simulink model "EngineCtrl_V1_1"  (R2018a)
settings: Solver=VariableStepAuto  StartTime=0.0  StopTime=10.0  FixedStep=sampletime  RelTol=1e-3  EnableMultiTasking=on
PreLoadFcn:
  | EngineCtrl_V1_BusInfo
libraries: simulink x2, simulink_extras x1
settings Model: Creator=IAEC nishito  LastModifiedBy=E00026
settings DataIOCC: LimitDataPoints=on  SaveFormat=Array  SignalLoggingSaveFormat=ModelDataLogs  SaveOutput=off  SaveTime=off
settings OptimizationCC: DefaultParameterBehavior=Inlined  ExpressionDepthLimit=2147483647  LifeSpan=inf
settings DebuggingCC: SolverPrmCheckMsg=warning  FcnCallInpInsideContextMsg=warning  StateNameClashWarn=warning  SFUnexpectedBacktrackingDiag=warning  SFNoUnconditionalDefaultTransitionDiag=warning  SFExecutionAtInitializationDiag=none
settings HardwareCC: ProdBitPerPointer=32  ProdBitPerSizeT=32  ProdBitPerPtrDiffT=32  ProdLargestAtomicFloat=None  ProdIntDivRoundTo=Undefined  ProdEndianess=Unspecified  ProdWordSize=32  ProdHWDeviceType=32-bit Generic
settings ModelReferenceCC: UpdateModelReferenceTargets=IfOutOfDate  PropagateSignalLabelsOutOfModel=off
settings CodeAppCC: StateflowObjectComments=on
settings GRTTargetCC: TargetLangStandard=C89/C90 (ANSI)  GeneratePreprocessorConditionals=Disable all  CombineOutputUpdateFcns=off  GRTInterface=on
settings ConfigComp: CovMetricSettings=dw  CovHtmlReporting=on  CovSaveCumulativeToWorkspaceVar=on  CovSaveSingleToWorkspaceVar=on  CovExternalEMLEnable=off

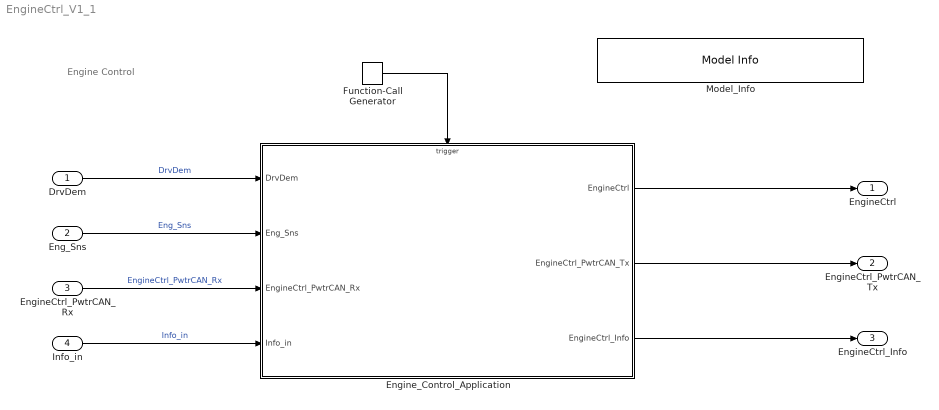
== system EngineCtrl_V1_1 ==
  note: Engine Control
  DrvDem : Inport  OutDataTypeStr=Bus: Driver_demand_Bus
      settings: AttributesFormatString=%<OutDataTypeStr>
  Eng_Sns : Inport  Port=2  OutDataTypeStr=Bus: Engine_sensor_Bus
      settings: AttributesFormatString=%<OutDataTypeStr>
  EngineCtrl_PwtrCAN_Rx : Inport  Port=3  OutDataTypeStr=Bus: EngineCtrl_PwtrCAN_Rx_Bus
      settings: AttributesFormatString=<%<OutDataTypeStr>>
  Info_in : Inport  Port=4  OutDataTypeStr=Bus: EngineCtrl_Info_in_Bus
      settings: AttributesFormatString=%<OutDataTypeStr>
  Engine_Control_Application : Subsystem
  Function-Call Generator : simulink/Ports & Subsystems/Function-Call Generator  sample_time=0.01  numberOfIterations=1
      settings: AttributesFormatString=<sample_time=%<sample_time>>
  Model_Info : simulink/Model-Wide Utilities/Model Info  Frame=on  DisplayStringWithTags=|  HorizontalTextAlignment=Left  LeftAlignmentValue=0.02
      | Version  %<ModelVersion>
      | LastModifided by %<LastModifiedBy>  Date %<LastModificationDate>
      | Description  %<Description>
  EngineCtrl : Outport  OutDataTypeStr=Bus: EngineCtrl_Bus
      settings: AttributesFormatString=<%<OutDataTypeStr>>
  EngineCtrl_PwtrCAN_Tx : Outport  Port=2  OutDataTypeStr=Bus: EngineCtrl_PwtrCAN_Tx_Bus
      settings: AttributesFormatString=<%<OutDataTypeStr>>
  EngineCtrl_Info : Outport  Port=3  OutDataTypeStr=Bus: EngineCtrl_Info_Bus
      settings: AttributesFormatString=<%<OutDataTypeStr>>
  wires:
  EngineCtrl_PwtrCAN_Rx/1 -> Engine_Control_Application/3(EngineCtrl_PwtrCAN_Rx)  "EngineCtrl_PwtrCAN_Rx"
  DrvDem/1 -> Engine_Control_Application/1(DrvDem)  "DrvDem"
  Eng_Sns/1 -> Engine_Control_Application/2(Eng_Sns)  "Eng_Sns"
  Function-Call Generator/1 -> Engine_Control_Application/Trigger
  Engine_Control_Application/2(EngineCtrl_PwtrCAN_Tx) -> EngineCtrl_PwtrCAN_Tx/1
  Engine_Control_Application/1(EngineCtrl) -> EngineCtrl/1
  Engine_Control_Application/3(EngineCtrl_Info) -> EngineCtrl_Info/1
  Info_in/1 -> Engine_Control_Application/4(Info_in)  "Info_in"

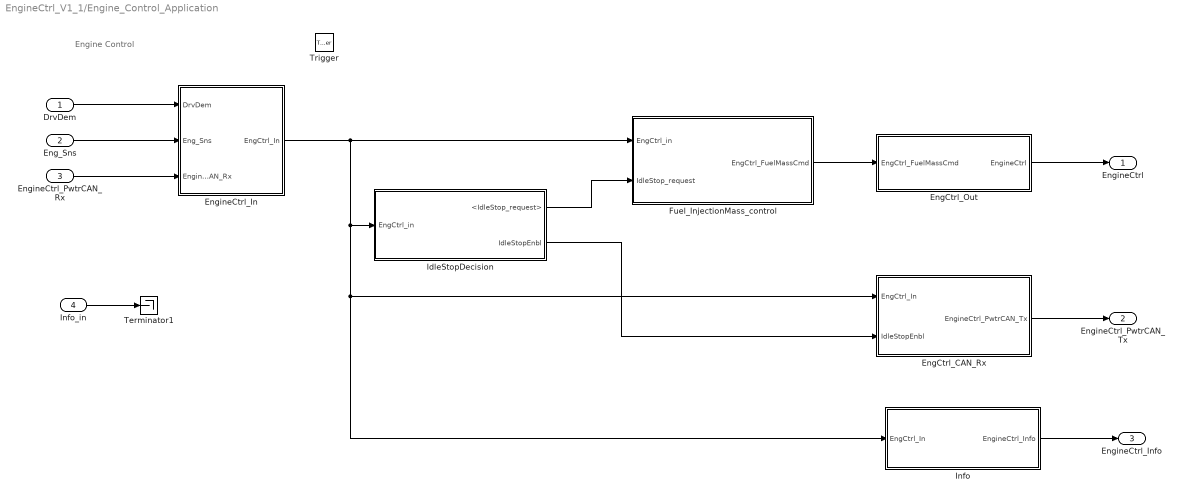
== system EngineCtrl_V1_1/Engine_Control_Application ==
  note: Engine Control
  DrvDem : Inport
  Eng_Sns : Inport  Port=2
  EngineCtrl_PwtrCAN_Rx : Inport  Port=3
  Info_in : Inport  Port=4
  Trigger : TriggerPort  TriggerType=function-call  VariantControl=Variant  PortDimensions=1
  EngCtrl_CAN_Rx : Subsystem
  EngCtrl_Out : Subsystem
  EngineCtrl_In : Subsystem
  Fuel_InjectionMass_control : Subsystem
  IdleStopDecision : Subsystem
  Info : Subsystem
  Terminator1 : Terminator
  EngineCtrl : Outport
  EngineCtrl_PwtrCAN_Tx : Outport  Port=2
  EngineCtrl_Info : Outport  Port=3
  wires:
  DrvDem/1 -> EngineCtrl_In/1(DrvDem)
  Info_in/1 -> Terminator1/1
  EngCtrl_CAN_Rx/1(EngineCtrl_PwtrCAN_Tx) -> EngineCtrl_PwtrCAN_Tx/1
  IdleStopDecision/2(IdleStopEnbl) -> EngCtrl_CAN_Rx/2(IdleStopEnbl)
  Eng_Sns/1 -> EngineCtrl_In/2(Eng_Sns)
  EngineCtrl_PwtrCAN_Rx/1 -> EngineCtrl_In/3(EngineCtrl_PwtrCAN_Rx)
  EngineCtrl_In/1(EngCtrl_In) -> Info/1(EngCtrl_In), EngCtrl_CAN_Rx/1(EngCtrl_In), IdleStopDecision/1(EngCtrl_in), Fuel_InjectionMass_control/1(EngCtrl_in)
  Info/1(EngineCtrl_Info) -> EngineCtrl_Info/1
  Fuel_InjectionMass_control/1(EngCtrl_FuelMassCmd) -> EngCtrl_Out/1(EngCtrl_FuelMassCmd)
  EngCtrl_Out/1(EngineCtrl) -> EngineCtrl/1
  IdleStopDecision/1(<IdleStop_request>) -> Fuel_InjectionMass_control/2(IdleStop_request)

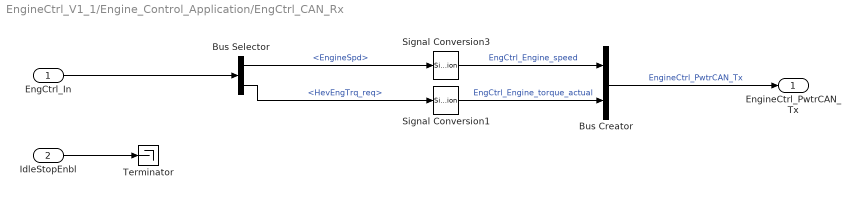
== system EngineCtrl_V1_1/Engine_Control_Application/EngCtrl_CAN_Rx ==
  EngCtrl_In : Inport
  IdleStopEnbl : Inport  Port=2
  Bus Creator : BusCreator  Inputs=2  OutDataTypeStr=Bus: EngineCtrl_PwtrCAN_Tx_Bus
      settings: AttributesFormatString=%<OutDataTypeStr>
  Bus Selector : BusSelector  OutputSignals=EngineSpd,HevEngTrq_req
  Signal Conversion1 : SignalConversion  OverrideOpt=off
  Signal Conversion3 : SignalConversion  OverrideOpt=off
  Terminator : Terminator
  EngineCtrl_PwtrCAN_Tx : Outport
  wires:
  Bus Creator/1 -> EngineCtrl_PwtrCAN_Tx/1  "EngineCtrl_PwtrCAN_Tx"
  Signal Conversion3/1 -> Bus Creator/1  "EngCtrl_Engine_speed"
  Signal Conversion1/1 -> Bus Creator/2  "EngCtrl_Engine_torque_actual"
  EngCtrl_In/1 -> Bus Selector/1
  Bus Selector/1 -> Signal Conversion3/1  "<EngineSpd>"
  Bus Selector/2 -> Signal Conversion1/1  "<HevEngTrq_req>"
  IdleStopEnbl/1 -> Terminator/1

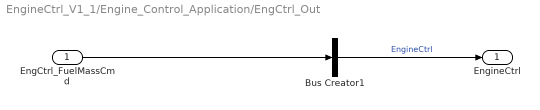
== system EngineCtrl_V1_1/Engine_Control_Application/EngCtrl_Out ==
  EngCtrl_FuelMassCmd : Inport
  Bus Creator1 : BusCreator  Inputs=1  OutDataTypeStr=Bus: EngineCtrl_Bus
      settings: AttributesFormatString=%<OutDataTypeStr>
  EngineCtrl : Outport
  wires:
  Bus Creator1/1 -> EngineCtrl/1  "EngineCtrl"
  EngCtrl_FuelMassCmd/1 -> Bus Creator1/1

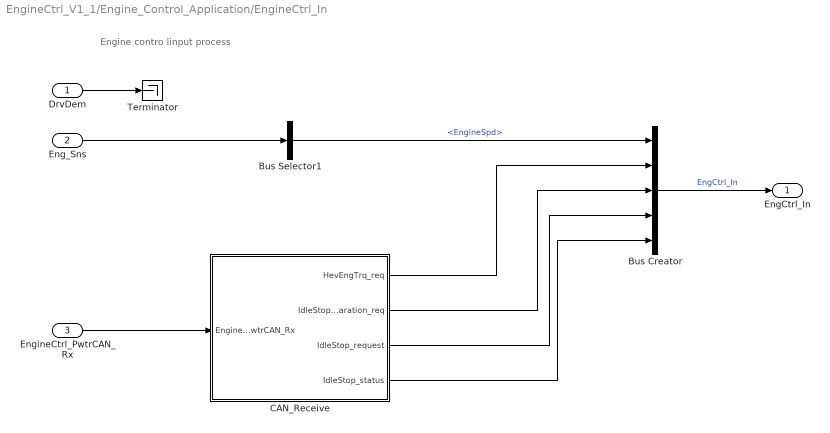
== system EngineCtrl_V1_1/Engine_Control_Application/EngineCtrl_In ==
  note: Engine contro linput process
  DrvDem : Inport
  Eng_Sns : Inport  Port=2
  EngineCtrl_PwtrCAN_Rx : Inport  Port=3
  Bus Creator : BusCreator  Inputs=5
  Bus Selector1 : BusSelector  OutputSignals=EngineSpd
  CAN_Receive : Subsystem
  Terminator : Terminator
  EngCtrl_In : Outport
  wires:
  EngineCtrl_PwtrCAN_Rx/1 -> CAN_Receive/1(EngineCtrl_PwtrCAN_Rx)
  Eng_Sns/1 -> Bus Selector1/1
  Bus Selector1/1 -> Bus Creator/1  "<EngineSpd>"
  CAN_Receive/1(HevEngTrq_req) -> Bus Creator/2
  CAN_Receive/4(IdleStop_status) -> Bus Creator/5
  CAN_Receive/2(IdleStop_preparation_req) -> Bus Creator/3
  CAN_Receive/3(IdleStop_request) -> Bus Creator/4
  Bus Creator/1 -> EngCtrl_In/1  "EngCtrl_In"
  DrvDem/1 -> Terminator/1

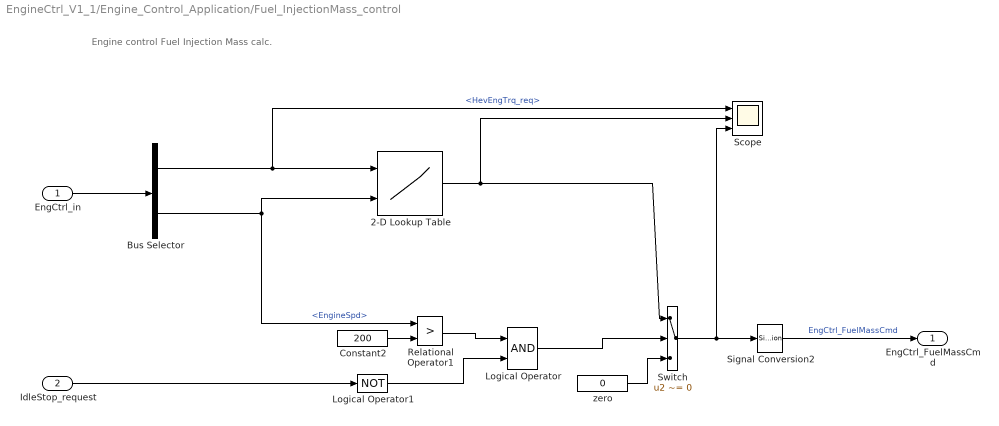
== system EngineCtrl_V1_1/Engine_Control_Application/Fuel_InjectionMass_control ==
  note: Engine control Fuel Injection Mass calc.
  EngCtrl_in : Inport
  IdleStop_request : Inport  Port=2
  2-D Lookup Table : Lookup_n-D  BreakpointsForDimension1=[0 400]  BreakpointsForDimension2=[0 200 600 1000]  Table=[0 10 0 0; 70 70 70 70]  InternalRulePriority=Speed  RndMeth=Simplest  InputSameDT=on
  Bus Selector : BusSelector  OutputSignals=HevEngTrq_req,EngineSpd
  Constant2 : Constant  Value=200
  Logical Operator : Logic  AllPortsSameDT=off  OutDataTypeStr=boolean
  Logical Operator1 : Logic  Operator=NOT  AllPortsSameDT=off  OutDataTypeStr=boolean
  Relational Operator1 : RelationalOperator  Operator=>  OutDataTypeStr=boolean  RndMeth=Nearest
  Scope : Scope  NumInputPorts=3
  Signal Conversion2 : SignalConversion  OverrideOpt=off
  Switch : Switch  Criteria=u2 ~= 0  Threshold=0.5  SaturateOnIntegerOverflow=on
      settings: AttributesFormatString=<%<Criteria>>
  zero : Constant  Value=0
  EngCtrl_FuelMassCmd : Outport
  wires:
  Switch/1 -> Scope/3, Signal Conversion2/1
  2-D Lookup Table/1 -> Switch/1, Scope/2
  Logical Operator1/1 -> Logical Operator/2
  Logical Operator/1 -> Switch/2
  zero/1 -> Switch/3
  Constant2/1 -> Relational Operator1/2
  Relational Operator1/1 -> Logical Operator/1
  Signal Conversion2/1 -> EngCtrl_FuelMassCmd/1  "EngCtrl_FuelMassCmd"
  EngCtrl_in/1 -> Bus Selector/1
  Bus Selector/1 -> Scope/1, 2-D Lookup Table/1  "<HevEngTrq_req>"
  Bus Selector/2 -> Relational Operator1/1, 2-D Lookup Table/2  "<EngineSpd>"
  IdleStop_request/1 -> Logical Operator1/1

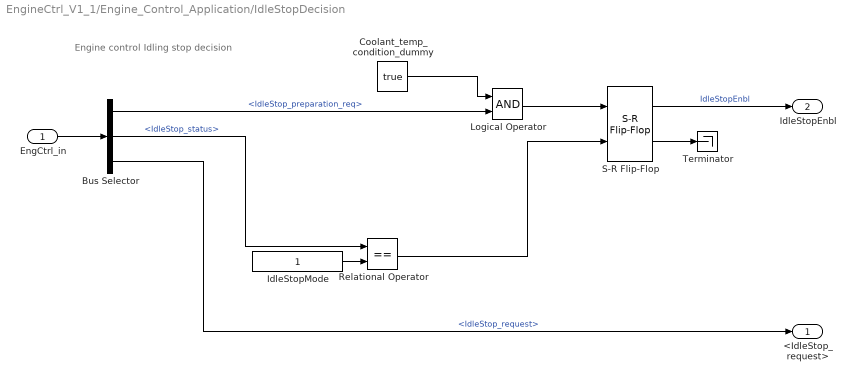
== system EngineCtrl_V1_1/Engine_Control_Application/IdleStopDecision ==
  note: Engine control Idling stop decision
  EngCtrl_in : Inport
  Bus Selector : BusSelector  OutputSignals=IdleStop_preparation_req,IdleStop_status,IdleStop_request
  Coolant_temp_condition_dummy : Constant  Value=true
  IdleStopMode : Constant  VectorParams1D=off  SampleTime=-1
  Logical Operator : Logic  AllPortsSameDT=off  OutDataTypeStr=boolean
  Relational Operator : RelationalOperator  Operator===  OutDataTypeStr=boolean  RndMeth=Simplest
  S-R Flip-Flop : simulink_extras/Flip Flops/S-R Flip-Flop  initial_condition=0
  Terminator : Terminator
  <IdleStop_request> : Outport
  IdleStopEnbl : Outport  Port=2
  wires:
  Coolant_temp_condition_dummy/1 -> Logical Operator/1
  Logical Operator/1 -> S-R Flip-Flop/1
  S-R Flip-Flop/2 -> Terminator/1
  S-R Flip-Flop/1 -> IdleStopEnbl/1  "IdleStopEnbl"
  EngCtrl_in/1 -> Bus Selector/1
  Bus Selector/1 -> Logical Operator/2  "<IdleStop_preparation_req>"
  Bus Selector/2 -> Relational Operator/1  "<IdleStop_status>"
  IdleStopMode/1 -> Relational Operator/2
  Relational Operator/1 -> S-R Flip-Flop/2
  Bus Selector/3 -> <IdleStop_request>/1  "<IdleStop_request>"

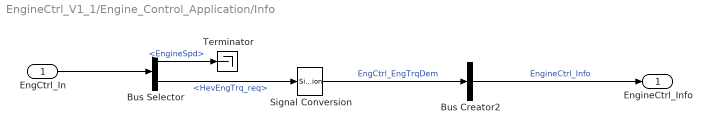
== system EngineCtrl_V1_1/Engine_Control_Application/Info ==
  EngCtrl_In : Inport
  Bus Creator2 : BusCreator  Inputs=1  OutDataTypeStr=Bus: EngineCtrl_Info_Bus
      settings: AttributesFormatString=%<OutDataTypeStr>
  Bus Selector : BusSelector  OutputSignals=EngineSpd,HevEngTrq_req
  Signal Conversion : SignalConversion  OverrideOpt=off
  Terminator : Terminator
  EngineCtrl_Info : Outport
  wires:
  Signal Conversion/1 -> Bus Creator2/1  "EngCtrl_EngTrqDem"
  Bus Creator2/1 -> EngineCtrl_Info/1  "EngineCtrl_Info"
  EngCtrl_In/1 -> Bus Selector/1
  Bus Selector/2 -> Signal Conversion/1  "<HevEngTrq_req>"
  Bus Selector/1 -> Terminator/1  "<EngineSpd>"

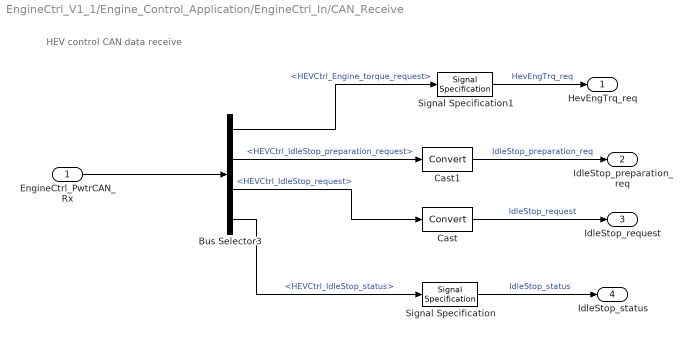
== system EngineCtrl_V1_1/Engine_Control_Application/EngineCtrl_In/CAN_Receive ==
  note: HEV control CAN data receive
  EngineCtrl_PwtrCAN_Rx : Inport
  Bus Selector3 : BusSelector  OutputSignals=HEVCtrl_Engine_torque_request,HEVCtrl_IdleStop_preparation_request,HEVCtrl_IdleStop_request,HEVCtrl_IdleStop_status
  Cast : DataTypeConversion
  Cast1 : DataTypeConversion
  Signal Specification : SignalSpecification
  Signal Specification1 : SignalSpecification
  HevEngTrq_req : Outport
  IdleStop_preparation_req : Outport  Port=2
  IdleStop_request : Outport  Port=3
  IdleStop_status : Outport  Port=4
  wires:
  Bus Selector3/1 -> Signal Specification1/1  "<HEVCtrl_Engine_torque_request>"
  Bus Selector3/2 -> Cast1/1  "<HEVCtrl_IdleStop_preparation_request>"
  Bus Selector3/3 -> Cast/1  "<HEVCtrl_IdleStop_request>"
  EngineCtrl_PwtrCAN_Rx/1 -> Bus Selector3/1
  Cast/1 -> IdleStop_request/1  "IdleStop_request"
  Cast1/1 -> IdleStop_preparation_req/1  "IdleStop_preparation_req"
  Bus Selector3/4 -> Signal Specification/1  "<HEVCtrl_IdleStop_status>"
  Signal Specification/1 -> IdleStop_status/1  "IdleStop_status"
  Signal Specification1/1 -> HevEngTrq_req/1  "HevEngTrq_req"
